simulink model "ALFlight3Wing"  (R2019a)
settings: Solver=VariableStepAuto  StartTime=0.0  StopTime=100  RelTol=1e-3
InitFcn:
  | Ts=.05
  | load('goodMPC.mat')
  | %load('fault2mpc.mat')
  | global counts
  | counts=0
  | 
  | An=[-0.0220400000000000,0.00142200000000000,0,-32.1700000000000,0,0,0,0,0,0;-0.0575900000000000,-0.394300000000000,871,0,0,0,0,0,0,0;-9.50000000000000e-05,-0.00179300000000000,-0.546800000000000,0,0,0,0,0,0,0;0,0,1,0,0,0,0,0,0,0;0,0,0,0,-0.0639900000000000,0,-1,0.0369100000000000,0,0;0,0,0,0,-2.11100000000000,-0.504800000000000,0.193000000000000,0,0,0;0,0,0,0,0.773200000000000,0.0108700000000000,-0.179400000000000,0,0,0;0,0,0,0,0,1,0,0,0,0;0,0,0,0,0,0,1,0,0,0;0,1,0,0,0,0,0,0,0,0]
  | Bn=[0,1.91000000000000e-05,0,0;-18.5800000000000,0,0,0;-1.20000000000000,0,0,0;0,0,0,0;0,0,0,0.00839000000000000;0,0,0.184800000000000,0.105600000000000;0,0,-0.00869900000000000,-0.459100000000000;0,0,0,0;0,0,0,0;0,0,0,0]
  | 
  | 
  |  set_param('ALFlight3Wing/ConstantA','Value','An')
  |  set_param('ALFlight3Wing/ConstantB','Value','Bn')
model workspace (MAT data in the model file):
  MCOS : class17 (value not decoded)
values from neighbouring files (symbols this model uses):
  Af2 = [-0.02204 -0.05759 -9.5e-05 0 0 0 0 0 0 0 0.001422 -0.3943 ... (100 elements, 10x10)]    [UpdatedWorkspace.mat]    (also in current2.mat; finalWorkspace.mat)
  Bf2 = [0 -18.58 -1.2 0 0 0 0 0 0 0 1.91e-05 0 ... (40 elements, 10x4)]    [UpdatedWorkspace.mat]    (also in current2.mat; finalWorkspace.mat)
  Cn = [1 0 0 0 0 0 0 0 0 0 0 0 ... (40 elements, 4x10)]    [UpdatedWorkspace.mat]    (also in current2.mat; finalWorkspace.mat)
  Dn = [0 0 0 0 0 0 0 0 0 0 0 0 ... (16 elements, 4x4)]    [UpdatedWorkspace.mat]    (also in current2.mat; finalWorkspace.mat)
  p = 15    [calcVar.m]    (also in chanceConstraintProgramming4.m = [norminv(.505),norminv(.6),norminv(.7),norminv(.8),norminv(.; dynamicsEst.m)
undefined symbols (not defined in the file or in its folder): Earth, iA, lastPcov, lastu, lastx, MDscale, mmpc_mvseq, mmpc_state, mmpc_ts, mmpc_u0, mmpc_xseq, mmpc_yseq, MVscale, nCC, nu, nud, nv, ny, nym, RMVscale, RYscale, ts, uoff, WGS84, xoff, Yscale
libraries: mpcsigdimcheck_private x44, simulink_extras x3, mpclib x2, commchan3 x1, aerolibtransform2 x1, aerolibfltsims x1, aerolibanimutils x1
(part 2 of 4)

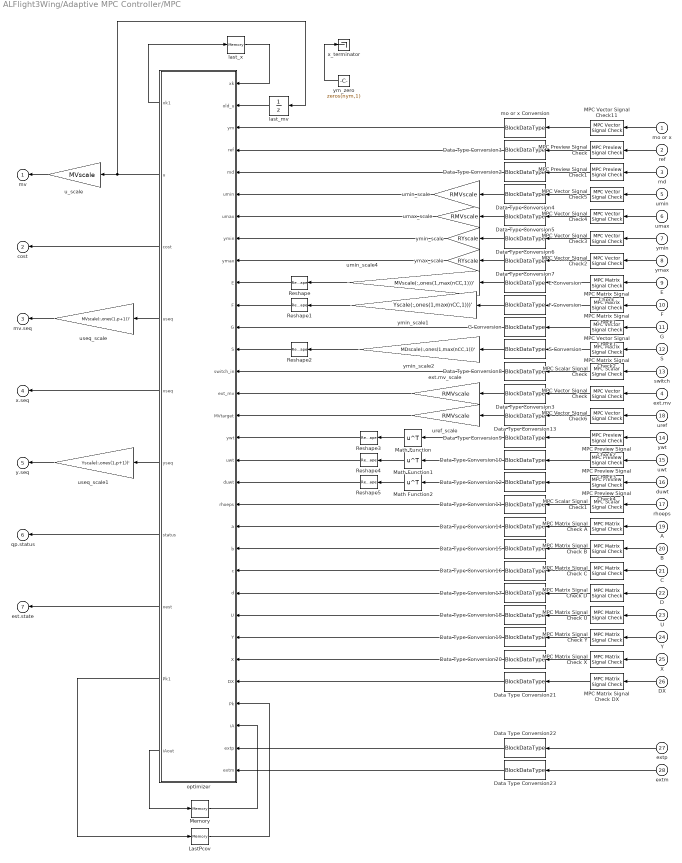
== system ALFlight3Wing/Adaptive MPC Controller/MPC ==
  mo or x : Inport
  ref : Inport  Port=2
  md : Inport  Port=3
  ext.mv : Inport  Port=4
  umin : Inport  Port=5
  umax : Inport  Port=6
  ymin : Inport  Port=7
  ymax : Inport  Port=8
  E : Inport  Port=9
  F : Inport  Port=10
  G : Inport  Port=11
  S : Inport  Port=12
  switch : Inport  Port=13
  ywt : Inport  Port=14
  uwt : Inport  Port=15
  duwt : Inport  Port=16
  rhoeps : Inport  Port=17
  uref : Inport  Port=18
  A : Inport  Port=19
  B : Inport  Port=20
  C : Inport  Port=21
  D : Inport  Port=22
  U : Inport  Port=23
  Y : Inport  Port=24
  X : Inport  Port=25
  DX : Inport  Port=26
  extp : Inport  Port=27
  extm : Inport  Port=28
  Data Type Conversion{1..23} (23 alike) : DataTypeConversion  OutDataTypeStr=BlockDataType
  E Conversion : DataTypeConversion  OutDataTypeStr=BlockDataType
  F Conversion : DataTypeConversion  OutDataTypeStr=BlockDataType
  G Conversion : DataTypeConversion  OutDataTypeStr=BlockDataType
  LastPcov : Memory  InitialCondition=lastPcov  InheritSampleTime=on  LinearizeAsDelay=on
  MPC Matrix Signal Check : mpcsigdimcheck_private/MPC Matrix Signal Check  blockname=blk  signalname='CustomConstraint.E'  numrow=max(nCC,1)  numcol=nu  steps=0  isLTV=0
      settings: SourceProductName=MATLAB Runtime - Model Predictive Control Toolbox Addin  SourceProductBaseCode=Missing
  MPC Matrix Signal Check A : mpcsigdimcheck_private/MPC Matrix Signal Check  blockname=blk  signalname='Model.A'  numrow=nxp  numcol=nxp  steps=p  isLTV=isLTV
      settings: SourceProductName=MATLAB Runtime - Model Predictive Control Toolbox Addin  SourceProductBaseCode=Missing
  MPC Matrix Signal Check B : mpcsigdimcheck_private/MPC Matrix Signal Check  blockname=blk  signalname='Model.B'  numrow=nxp  numcol=nu+nv-1+nud  steps=p  isLTV=isLTV
      settings: SourceProductName=MATLAB Runtime - Model Predictive Control Toolbox Addin  SourceProductBaseCode=Missing
  MPC Matrix Signal Check C : mpcsigdimcheck_private/MPC Matrix Signal Check  blockname=blk  signalname='Model.C'  numrow=ny  numcol=nxp  steps=p  isLTV=isLTV
      settings: SourceProductName=MATLAB Runtime - Model Predictive Control Toolbox Addin  SourceProductBaseCode=Missing
  MPC Matrix Signal Check D : mpcsigdimcheck_private/MPC Matrix Signal Check  blockname=blk  signalname='Model.D'  numrow=ny  numcol=nu+nv-1+nud  steps=p  isLTV=isLTV
      settings: SourceProductName=MATLAB Runtime - Model Predictive Control Toolbox Addin  SourceProductBaseCode=Missing
  MPC Matrix Signal Check DX : mpcsigdimcheck_private/MPC Matrix Signal Check  blockname=blk  signalname='Model.DX'  numrow=nxp  numcol=1  steps=p  isLTV=isLTV
      settings: SourceProductName=MATLAB Runtime - Model Predictive Control Toolbox Addin  SourceProductBaseCode=Missing
  MPC Matrix Signal Check U : mpcsigdimcheck_private/MPC Matrix Signal Check  blockname=blk  signalname='Model.U'  numrow=nu+nv-1+nud  numcol=1  steps=p  isLTV=isLTV
      settings: SourceProductName=MATLAB Runtime - Model Predictive Control Toolbox Addin  SourceProductBaseCode=Missing
  MPC Matrix Signal Check X : mpcsigdimcheck_private/MPC Matrix Signal Check  blockname=blk  signalname='Model.X'  numrow=nxp  numcol=1  steps=p  isLTV=isLTV
      settings: SourceProductName=MATLAB Runtime - Model Predictive Control Toolbox Addin  SourceProductBaseCode=Missing
  MPC Matrix Signal Check Y : mpcsigdimcheck_private/MPC Matrix Signal Check  blockname=blk  signalname='Model.Y'  numrow=ny  numcol=1  steps=p  isLTV=isLTV
      settings: SourceProductName=MATLAB Runtime - Model Predictive Control Toolbox Addin  SourceProductBaseCode=Missing
  MPC Matrix Signal Check1 : mpcsigdimcheck_private/MPC Matrix Signal Check  blockname=blk  signalname='CustomConstraint.F'  numrow=max(nCC,1)  numcol=ny  steps=0  isLTV=0
      settings: SourceProductName=MATLAB Runtime - Model Predictive Control Toolbox Addin  SourceProductBaseCode=Missing
  MPC Matrix Signal Check2 : mpcsigdimcheck_private/MPC Matrix Signal Check  blockname=blk  signalname='CustomConstraint.S'  numrow=max(nCC,1)  numcol=max(nv-1,1)  steps=0  isLTV=0
      settings: SourceProductName=MATLAB Runtime - Model Predictive Control Toolbox Addin  SourceProductBaseCode=Missing
  MPC Preview Signal Check : mpcsigdimcheck_private/MPC Preview Signal Check  blockname=blk  signalname='ref'  numrow=p  numcol=ny
      settings: SourceProductName=MATLAB Runtime - Model Predictive Control Toolbox Addin  SourceProductBaseCode=Missing
  MPC Preview Signal Check1 : mpcsigdimcheck_private/MPC Preview Signal Check  blockname=blk  signalname='md'  numrow=p+1  numcol=max(nv-1,1)
      settings: SourceProductName=MATLAB Runtime - Model Predictive Control Toolbox Addin  SourceProductBaseCode=Missing
  MPC Preview Signal Check2 : mpcsigdimcheck_private/MPC Preview Signal Check  blockname=blk  signalname='y.wt'  numrow=p  numcol=ny
      settings: SourceProductName=MATLAB Runtime - Model Predictive Control Toolbox Addin  SourceProductBaseCode=Missing
  MPC Preview Signal Check3 : mpcsigdimcheck_private/MPC Preview Signal Check  blockname=blk  signalname='u.wt'  numrow=p  numcol=nu
      settings: SourceProductName=MATLAB Runtime - Model Predictive Control Toolbox Addin  SourceProductBaseCode=Missing
  MPC Preview Signal Check4 : mpcsigdimcheck_private/MPC Preview Signal Check  blockname=blk  signalname='du.wt'  numrow=p  numcol=nu
      settings: SourceProductName=MATLAB Runtime - Model Predictive Control Toolbox Addin  SourceProductBaseCode=Missing
  MPC Scalar Signal Check : mpcsigdimcheck_private/MPC Scalar Signal Check  blockname=blk  signalname='switch'
      settings: SourceProductName=MATLAB Runtime - Model Predictive Control Toolbox Addin  SourceProductBaseCode=Missing
  MPC Scalar Signal Check1 : mpcsigdimcheck_private/MPC Scalar Signal Check  blockname=blk  signalname='ecr.wt'
      settings: SourceProductName=MATLAB Runtime - Model Predictive Control Toolbox Addin  SourceProductBaseCode=Missing
  MPC Vector Signal Check : mpcsigdimcheck_private/MPC Vector Signal Check  blockname=blk  signalname='ext.mv'  num=nu  vectortype=Any
      settings: SourceProductName=MATLAB Runtime - Model Predictive Control Toolbox Addin  SourceProductBaseCode=Missing
  MPC Vector Signal Check1 : mpcsigdimcheck_private/MPC Vector Signal Check  blockname=blk  signalname='CustomConstraint.G'  num=max(nCC,1)  vectortype=Column
      settings: SourceProductName=MATLAB Runtime - Model Predictive Control Toolbox Addin  SourceProductBaseCode=Missing
  MPC Vector Signal Check11 : mpcsigdimcheck_private/MPC Vector Signal Check  blockname=blk  signalname=strmoorx  num=nmoorx  vectortype=Any
      settings: SourceProductName=MATLAB Runtime - Model Predictive Control Toolbox Addin  SourceProductBaseCode=Missing
  MPC Vector Signal Check2 : mpcsigdimcheck_private/MPC Vector Signal Check  blockname=blk  signalname='ymax'  num=ny  vectortype=Any
      settings: SourceProductName=MATLAB Runtime - Model Predictive Control Toolbox Addin  SourceProductBaseCode=Missing
  MPC Vector Signal Check3 : mpcsigdimcheck_private/MPC Vector Signal Check  blockname=blk  signalname='ymin'  num=ny  vectortype=Any
      settings: SourceProductName=MATLAB Runtime - Model Predictive Control Toolbox Addin  SourceProductBaseCode=Missing
  MPC Vector Signal Check4 : mpcsigdimcheck_private/MPC Vector Signal Check  blockname=blk  signalname='umax'  num=nu  vectortype=Any
      settings: SourceProductName=MATLAB Runtime - Model Predictive Control Toolbox Addin  SourceProductBaseCode=Missing
  MPC Vector Signal Check5 : mpcsigdimcheck_private/MPC Vector Signal Check  blockname=blk  signalname='umin'  num=nu  vectortype=Any
      settings: SourceProductName=MATLAB Runtime - Model Predictive Control Toolbox Addin  SourceProductBaseCode=Missing
  MPC Vector Signal Check6 : mpcsigdimcheck_private/MPC Vector Signal Check  blockname=blk  signalname='mv.target'  num=nu  vectortype=Any
      settings: SourceProductName=MATLAB Runtime - Model Predictive Control Toolbox Addin  SourceProductBaseCode=Missing
  Math Function : Math  Operator=transpose  SaturateOnIntegerOverflow=on
  Math Function1 : Math  Operator=transpose  SaturateOnIntegerOverflow=on
  Math Function2 : Math  Operator=transpose  SaturateOnIntegerOverflow=on
  Memory : Memory  InitialCondition=iA  InheritSampleTime=on  LinearizeAsDelay=on
  Reshape : Reshape  OutputDimensionality=Customize  OutputDimensions=double([max(nCC,1),nu])
  Reshape1 : Reshape  OutputDimensionality=Customize  OutputDimensions=double([max(nCC,1),ny])
  Reshape2 : Reshape  OutputDimensionality=Customize  OutputDimensions=double([max(nCC,1),max(nv-1,1)])
  Reshape3 : Reshape  OutputDimensionality=Column vector (2-D)
  Reshape4 : Reshape  OutputDimensionality=Column vector (2-D)
  Reshape5 : Reshape  OutputDimensionality=Column vector (2-D)
  S Conversion : DataTypeConversion  OutDataTypeStr=BlockDataType
  ext.mv_scale : Gain  Gain=RMVscale  SampleTime=ts
  last_mv : UnitDelay  InitialCondition=lastu+uoff  SampleTime=ts  HasFrameUpgradeWarning=on
  last_x : Memory  InitialCondition=lastx+xoff  InheritSampleTime=on  LinearizeAsDelay=on
  mo or x Conversion : DataTypeConversion  OutDataTypeStr=BlockDataType
  optimizer : Subsystem  VariantControlMode=Label  Variant=on  VariantControl=Variant1  LabelModeActiveChoice=FixedHorizon
  u_scale : Gain  Gain=MVscale  SampleTime=ts
  umax_scale : Gain  Gain=RMVscale  SampleTime=ts
  umin_scale : Gain  Gain=RMVscale  SampleTime=ts
  umin_scale4 : Gain  Gain=MVscale(:,ones(1,max(nCC,1)))'  SampleTime=ts
  uref_scale : Gain  Gain=RMVscale  SampleTime=ts
  useq_scale : Gain  Gain=MVscale(:,ones(1,p+1))'  SampleTime=ts
  useq_scale1 : Gain  Gain=Yscale(:,ones(1,p+1))'  SampleTime=ts
  x_terminator : Terminator
  ym_zero : Constant  Value=zeros(nym,1)  OutDataTypeStr=BlockDataType
  ymax_scale : Gain  Gain=RYscale  SampleTime=ts
  ymin_scale : Gain  Gain=RYscale  SampleTime=ts
  ymin_scale1 : Gain  Gain=Yscale(:,ones(1,max(nCC,1)))'  SampleTime=ts
  ymin_scale2 : Gain  Gain=MDscale(:,ones(1,max(nCC,1)))'  SampleTime=ts
  mv : Outport  OutDataTypeStr=BlockDataType
  cost : Outport  Port=2  OutDataTypeStr=BlockDataType
  mv.seq : Outport  Port=3  OutDataTypeStr=BlockDataType
  x.seq : Outport  Port=4  OutDataTypeStr=BlockDataType
  y.seq : Outport  Port=5  OutDataTypeStr=BlockDataType
  qp.status : Outport  Port=6  OutDataTypeStr=BlockDataType
  est.state : Outport  Port=7  OutDataTypeStr=BlockDataType
  wires:
  extm/1 -> Data Type Conversion23/1
  extp/1 -> Data Type Conversion22/1
  Data Type Conversion23/1 -> optimizer/32(extm)
  Data Type Conversion22/1 -> optimizer/31(extp)
  optimizer/10(" iAout") -> Memory/1
  optimizer/9(" Pk1") -> LastPcov/1
  optimizer/8(" xest") -> est.state/1
  optimizer/7(" status") -> qp.status/1
  optimizer/6(" yseq") -> useq_scale1/1
  optimizer/5(" xseq") -> x.seq/1
  optimizer/4(" useq") -> useq_scale/1
  optimizer/3(" cost") -> cost/1
  optimizer/2(" u") -> last_mv/1, u_scale/1
  optimizer/1(" xk1") -> last_x/1
  Memory/1 -> optimizer/30("iA ")
  LastPcov/1 -> optimizer/29("Pk ")
  Data Type Conversion21/1 -> optimizer/28("DX ")
  Data Type Conversion20/1 -> optimizer/27("X ")
  Data Type Conversion19/1 -> optimizer/26("Y ")
  Data Type Conversion18/1 -> optimizer/25("U ")
  Data Type Conversion17/1 -> optimizer/24("d ")
  Data Type Conversion16/1 -> optimizer/23("c ")
  Data Type Conversion15/1 -> optimizer/22("b ")
  Data Type Conversion14/1 -> optimizer/21("a ")
  Data Type Conversion11/1 -> optimizer/20("rhoeps ")
  Reshape5/1 -> optimizer/19("duwt ")
  Reshape4/1 -> optimizer/18("uwt ")
  Reshape3/1 -> optimizer/17("ywt ")
  uref_scale/1 -> optimizer/16("MVtarget ")
  ext.mv_scale/1 -> optimizer/15("ext_mv ")
  Data Type Conversion8/1 -> optimizer/14("switch_in ")
  Reshape2/1 -> optimizer/13("S ")
  G Conversion/1 -> optimizer/12("G ")
  Reshape1/1 -> optimizer/11("F ")
  Reshape/1 -> optimizer/10("E ")
  ymax_scale/1 -> optimizer/9("ymax ")
  ymin_scale/1 -> optimizer/8("ymin ")
  umax_scale/1 -> optimizer/7("umax ")
  umin_scale/1 -> optimizer/6("umin ")
  Data Type Conversion2/1 -> optimizer/5("md ")
  Data Type Conversion1/1 -> optimizer/4("ref ")
  mo or x Conversion/1 -> optimizer/3("ym ")
  last_mv/1 -> optimizer/2("old_u ")
  last_x/1 -> optimizer/1("xk ")
  useq_scale1/1 -> y.seq/1
  Math Function2/1 -> Reshape5/1
  Math Function1/1 -> Reshape4/1
  Math Function/1 -> Reshape3/1
  MPC Matrix Signal Check1/1 -> F Conversion/1
  umin_scale4/1 -> Reshape/1
  ymin_scale1/1 -> Reshape1/1
  G/1 -> MPC Vector Signal Check1/1
  F/1 -> MPC Matrix Signal Check1/1
  E Conversion/1 -> umin_scale4/1
  ymin_scale2/1 -> Reshape2/1
  MPC Matrix Signal Check/1 -> E Conversion/1
  S/1 -> MPC Matrix Signal Check2/1
  E/1 -> MPC Matrix Signal Check/1
  MPC Matrix Signal Check2/1 -> S Conversion/1
  MPC Vector Signal Check1/1 -> G Conversion/1
  S Conversion/1 -> ymin_scale2/1
  F Conversion/1 -> ymin_scale1/1
  MPC Matrix Signal Check DX/1 -> Data Type Conversion21/1
  MPC Matrix Signal Check X/1 -> Data Type Conversion20/1
  MPC Matrix Signal Check Y/1 -> Data Type Conversion19/1
  MPC Matrix Signal Check U/1 -> Data Type Conversion18/1
  MPC Matrix Signal Check D/1 -> Data Type Conversion17/1
  MPC Matrix Signal Check C/1 -> Data Type Conversion16/1
  MPC Matrix Signal Check B/1 -> Data Type Conversion15/1
  MPC Matrix Signal Check A/1 -> Data Type Conversion14/1
  MPC Scalar Signal Check1/1 -> Data Type Conversion11/1
  MPC Preview Signal Check4/1 -> Data Type Conversion12/1
  MPC Preview Signal Check3/1 -> Data Type Conversion10/1
  MPC Preview Signal Check2/1 -> Data Type Conversion9/1
  MPC Vector Signal Check6/1 -> Data Type Conversion13/1
  MPC Vector Signal Check/1 -> Data Type Conversion3/1
  MPC Scalar Signal Check/1 -> Data Type Conversion8/1
  MPC Vector Signal Check2/1 -> Data Type Conversion7/1
  MPC Vector Signal Check3/1 -> Data Type Conversion6/1
  MPC Vector Signal Check4/1 -> Data Type Conversion5/1
  MPC Vector Signal Check5/1 -> Data Type Conversion4/1
  MPC Preview Signal Check1/1 -> Data Type Conversion2/1
  MPC Preview Signal Check/1 -> Data Type Conversion1/1
  MPC Vector Signal Check11/1 -> mo or x Conversion/1
  useq_scale/1 -> mv.seq/1
  u_scale/1 -> mv/1
  DX/1 -> MPC Matrix Signal Check DX/1
  X/1 -> MPC Matrix Signal Check X/1
  Y/1 -> MPC Matrix Signal Check Y/1
  U/1 -> MPC Matrix Signal Check U/1
  D/1 -> MPC Matrix Signal Check D/1
  C/1 -> MPC Matrix Signal Check C/1
  B/1 -> MPC Matrix Signal Check B/1
  A/1 -> MPC Matrix Signal Check A/1
  md/1 -> MPC Preview Signal Check1/1
  umin/1 -> MPC Vector Signal Check5/1
  umax/1 -> MPC Vector Signal Check4/1
  ymin/1 -> MPC Vector Signal Check3/1
  ymax/1 -> MPC Vector Signal Check2/1
  switch/1 -> MPC Scalar Signal Check/1
  ext.mv/1 -> MPC Vector Signal Check/1
  Data Type Conversion3/1 -> ext.mv_scale/1
  ref/1 -> MPC Preview Signal Check/1
  mo or x/1 -> MPC Vector Signal Check11/1
  ywt/1 -> MPC Preview Signal Check2/1
  uwt/1 -> MPC Preview Signal Check3/1
  Data Type Conversion4/1 -> umin_scale/1
  Data Type Conversion5/1 -> umax_scale/1
  Data Type Conversion7/1 -> ymax_scale/1
  Data Type Conversion9/1 -> Math Function/1
  Data Type Conversion12/1 -> Math Function2/1
  Data Type Conversion6/1 -> ymin_scale/1
  rhoeps/1 -> MPC Scalar Signal Check1/1
  duwt/1 -> MPC Preview Signal Check4/1
  Data Type Conversion10/1 -> Math Function1/1
  uref/1 -> MPC Vector Signal Check6/1
  Data Type Conversion13/1 -> uref_scale/1
  ym_zero/1 -> x_terminator/1

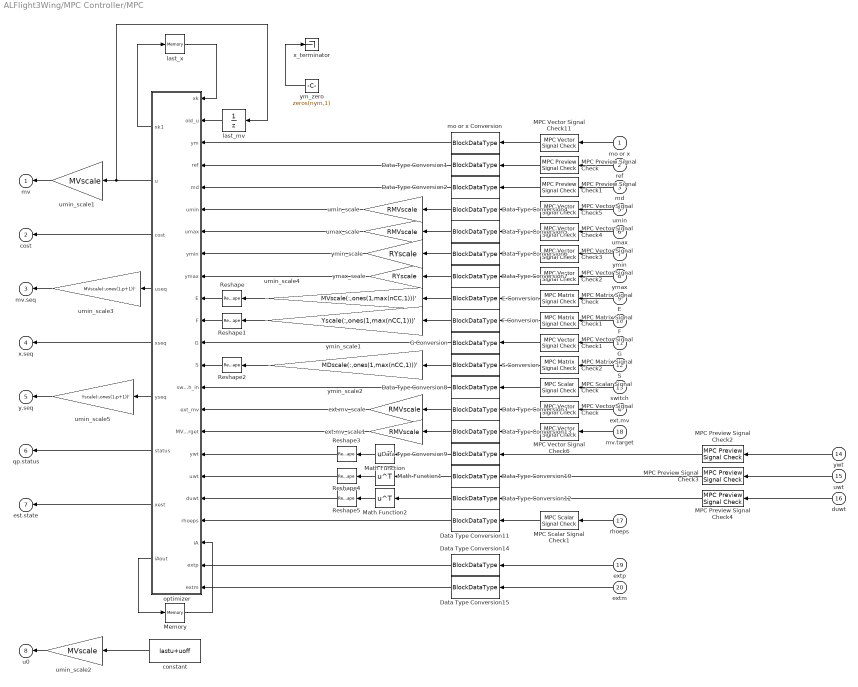
== system ALFlight3Wing/MPC Controller/MPC ==
  mo or x : Inport
  ref : Inport  Port=2
  md : Inport  Port=3
  ext.mv : Inport  Port=4
  umin : Inport  Port=5
  umax : Inport  Port=6
  ymin : Inport  Port=7
  ymax : Inport  Port=8
  E : Inport  Port=9
  F : Inport  Port=10
  G : Inport  Port=11
  S : Inport  Port=12
  switch : Inport  Port=13
  ywt : Inport  Port=14
  uwt : Inport  Port=15
  duwt : Inport  Port=16
  rhoeps : Inport  Port=17
  mv.target : Inport  Port=18
  extp : Inport  Port=19
  extm : Inport  Port=20
  Data Type Conversion{1..15} (15 alike) : DataTypeConversion  OutDataTypeStr=BlockDataType
  E Conversion : DataTypeConversion  OutDataTypeStr=BlockDataType
  F Conversion : DataTypeConversion  OutDataTypeStr=BlockDataType
  G Conversion : DataTypeConversion  OutDataTypeStr=BlockDataType
  MPC Matrix Signal Check : mpcsigdimcheck_private/MPC Matrix Signal Check  blockname=blk  signalname='CustomConstraint.E'  numrow=max(nCC,1)  numcol=nu  steps=0  isLTV=0
      settings: SourceProductName=MATLAB Runtime - Model Predictive Control Toolbox Addin  SourceProductBaseCode=Missing
  MPC Matrix Signal Check1 : mpcsigdimcheck_private/MPC Matrix Signal Check  blockname=blk  signalname='CustomConstraint.F'  numrow=max(nCC,1)  numcol=ny  steps=0  isLTV=0
      settings: SourceProductName=MATLAB Runtime - Model Predictive Control Toolbox Addin  SourceProductBaseCode=Missing
  MPC Matrix Signal Check2 : mpcsigdimcheck_private/MPC Matrix Signal Check  blockname=blk  signalname='CustomConstraint.S'  numrow=max(nCC,1)  numcol=max(nv-1,1)  steps=0  isLTV=0
      settings: SourceProductName=MATLAB Runtime - Model Predictive Control Toolbox Addin  SourceProductBaseCode=Missing
  MPC Preview Signal Check : mpcsigdimcheck_private/MPC Preview Signal Check  blockname=blk  signalname='ref'  numrow=p  numcol=ny
      settings: SourceProductName=MATLAB Runtime - Model Predictive Control Toolbox Addin  SourceProductBaseCode=Missing
  MPC Preview Signal Check1 : mpcsigdimcheck_private/MPC Preview Signal Check  blockname=blk  signalname='md'  numrow=p+1  numcol=max(nv-1,1)
      settings: SourceProductName=MATLAB Runtime - Model Predictive Control Toolbox Addin  SourceProductBaseCode=Missing
  MPC Preview Signal Check2 : mpcsigdimcheck_private/MPC Preview Signal Check  blockname=blk  signalname='y.wt'  numrow=p  numcol=ny
      settings: SourceProductName=MATLAB Runtime - Model Predictive Control Toolbox Addin  SourceProductBaseCode=Missing
  MPC Preview Signal Check3 : mpcsigdimcheck_private/MPC Preview Signal Check  blockname=blk  signalname='u.wt'  numrow=p  numcol=nu
      settings: SourceProductName=MATLAB Runtime - Model Predictive Control Toolbox Addin  SourceProductBaseCode=Missing
  MPC Preview Signal Check4 : mpcsigdimcheck_private/MPC Preview Signal Check  blockname=blk  signalname='du.wt'  numrow=p  numcol=nu
      settings: SourceProductName=MATLAB Runtime - Model Predictive Control Toolbox Addin  SourceProductBaseCode=Missing
  MPC Scalar Signal Check : mpcsigdimcheck_private/MPC Scalar Signal Check  blockname=blk  signalname='switch'
      settings: SourceProductName=MATLAB Runtime - Model Predictive Control Toolbox Addin  SourceProductBaseCode=Missing
  MPC Scalar Signal Check1 : mpcsigdimcheck_private/MPC Scalar Signal Check  blockname=blk  signalname='ecr.wt'
      settings: SourceProductName=MATLAB Runtime - Model Predictive Control Toolbox Addin  SourceProductBaseCode=Missing
  MPC Vector Signal Check : mpcsigdimcheck_private/MPC Vector Signal Check  blockname=blk  signalname='ext.mv'  num=nu  vectortype=Any
      settings: SourceProductName=MATLAB Runtime - Model Predictive Control Toolbox Addin  SourceProductBaseCode=Missing
  MPC Vector Signal Check1 : mpcsigdimcheck_private/MPC Vector Signal Check  blockname=blk  signalname='CustomConstraint.G'  num=max(nCC,1)  vectortype=Column
      settings: SourceProductName=MATLAB Runtime - Model Predictive Control Toolbox Addin  SourceProductBaseCode=Missing
  MPC Vector Signal Check11 : mpcsigdimcheck_private/MPC Vector Signal Check  blockname=blk  signalname=strmoorx  num=nmoorx  vectortype=Any
      settings: SourceProductName=MATLAB Runtime - Model Predictive Control Toolbox Addin  SourceProductBaseCode=Missing
  MPC Vector Signal Check2 : mpcsigdimcheck_private/MPC Vector Signal Check  blockname=blk  signalname='ymax'  num=ny  vectortype=Any
      settings: SourceProductName=MATLAB Runtime - Model Predictive Control Toolbox Addin  SourceProductBaseCode=Missing
  MPC Vector Signal Check3 : mpcsigdimcheck_private/MPC Vector Signal Check  blockname=blk  signalname='ymin'  num=ny  vectortype=Any
      settings: SourceProductName=MATLAB Runtime - Model Predictive Control Toolbox Addin  SourceProductBaseCode=Missing
  MPC Vector Signal Check4 : mpcsigdimcheck_private/MPC Vector Signal Check  blockname=blk  signalname='umax'  num=nu  vectortype=Any
      settings: SourceProductName=MATLAB Runtime - Model Predictive Control Toolbox Addin  SourceProductBaseCode=Missing
  MPC Vector Signal Check5 : mpcsigdimcheck_private/MPC Vector Signal Check  blockname=blk  signalname='umin'  num=nu  vectortype=Any
      settings: SourceProductName=MATLAB Runtime - Model Predictive Control Toolbox Addin  SourceProductBaseCode=Missing
  MPC Vector Signal Check6 : mpcsigdimcheck_private/MPC Vector Signal Check  blockname=blk  signalname='mv.target'  num=nu  vectortype=Any
      settings: SourceProductName=MATLAB Runtime - Model Predictive Control Toolbox Addin  SourceProductBaseCode=Missing
  Math Function : Math  Operator=transpose  SaturateOnIntegerOverflow=on
  Math Function1 : Math  Operator=transpose  SaturateOnIntegerOverflow=on
  Math Function2 : Math  Operator=transpose  SaturateOnIntegerOverflow=on
  Memory : Memory  InitialCondition=iA  InheritSampleTime=on  LinearizeAsDelay=on
  Reshape : Reshape  OutputDimensionality=Customize  OutputDimensions=double([max(nCC,1),nu])
  Reshape1 : Reshape  OutputDimensionality=Customize  OutputDimensions=double([max(nCC,1),ny])
  Reshape2 : Reshape  OutputDimensionality=Customize  OutputDimensions=double([max(nCC,1),max(nv-1,1)])
  Reshape3 : Reshape  OutputDimensionality=Column vector (2-D)
  Reshape4 : Reshape  OutputDimensionality=Column vector (2-D)
  Reshape5 : Reshape  OutputDimensionality=Column vector (2-D)
  S Conversion : DataTypeConversion  OutDataTypeStr=BlockDataType
  constant : Constant  Value=lastu+uoff
  ext.mv_scale : Gain  Gain=RMVscale  SampleTime=ts
  ext.mv_scale1 : Gain  Gain=RMVscale  SampleTime=ts
  last_mv : UnitDelay  InitialCondition=lastu+uoff  SampleTime=ts  HasFrameUpgradeWarning=on
  last_x : Memory  InitialCondition=lastx+xoff  InheritSampleTime=on  LinearizeAsDelay=on
  mo or x Conversion : DataTypeConversion  OutDataTypeStr=BlockDataType
  optimizer : Subsystem  VariantControlMode=Label  Variant=on  VariantControl=Variant1  LabelModeActiveChoice=FixedHorizon
  umax_scale : Gain  Gain=RMVscale  SampleTime=ts
  umin_scale : Gain  Gain=RMVscale  SampleTime=ts
  umin_scale1 : Gain  Gain=MVscale  SampleTime=ts
  umin_scale2 : Gain  Gain=MVscale  SampleTime=ts
  umin_scale3 : Gain  Gain=MVscale(:,ones(1,p+1))'  SampleTime=ts
  umin_scale4 : Gain  Gain=MVscale(:,ones(1,max(nCC,1)))'  SampleTime=ts
  umin_scale5 : Gain  Gain=Yscale(:,ones(1,p+1))'  SampleTime=ts
  x_terminator : Terminator
  ym_zero : Constant  Value=zeros(nym,1)  OutDataTypeStr=BlockDataType
  ymax_scale : Gain  Gain=RYscale  SampleTime=ts
  ymin_scale : Gain  Gain=RYscale  SampleTime=ts
  ymin_scale1 : Gain  Gain=Yscale(:,ones(1,max(nCC,1)))'  SampleTime=ts
  ymin_scale2 : Gain  Gain=MDscale(:,ones(1,max(nCC,1)))'  SampleTime=ts
  mv : Outport  OutDataTypeStr=BlockDataType
  cost : Outport  Port=2  OutDataTypeStr=BlockDataType
  mv.seq : Outport  Port=3  OutDataTypeStr=BlockDataType
  x.seq : Outport  Port=4  OutDataTypeStr=BlockDataType
  y.seq : Outport  Port=5  OutDataTypeStr=BlockDataType
  qp.status : Outport  Port=6  OutDataTypeStr=BlockDataType
  est.state : Outport  Port=7  OutDataTypeStr=BlockDataType
  u0 : Outport  Port=8  OutDataTypeStr=BlockDataType
  wires:
  extm/1 -> Data Type Conversion15/1
  extp/1 -> Data Type Conversion14/1
  Data Type Conversion14/1 -> optimizer/22(extp)
  Data Type Conversion15/1 -> optimizer/23(extm)
  optimizer/9(" iAout") -> Memory/1
  optimizer/8(" xest") -> est.state/1
  optimizer/7(" status") -> qp.status/1
  optimizer/6(" yseq") -> umin_scale5/1
  optimizer/5(" xseq") -> x.seq/1
  optimizer/4(" useq") -> umin_scale3/1
  optimizer/3(" cost") -> cost/1
  optimizer/2(" u") -> umin_scale1/1, last_mv/1
  optimizer/1(" xk1") -> last_x/1
  Memory/1 -> optimizer/21("iA ")
  Data Type Conversion11/1 -> optimizer/20("rhoeps ")
  Reshape5/1 -> optimizer/19("duwt ")
  Reshape4/1 -> optimizer/18("uwt ")
  Reshape3/1 -> optimizer/17("ywt ")
  ext.mv_scale1/1 -> optimizer/16("MVtarget ")
  ext.mv_scale/1 -> optimizer/15("ext_mv ")
  Data Type Conversion8/1 -> optimizer/14("switch_in ")
  Reshape2/1 -> optimizer/13("S ")
  G Conversion/1 -> optimizer/12("G ")
  Reshape1/1 -> optimizer/11("F ")
  Reshape/1 -> optimizer/10("E ")
  ymax_scale/1 -> optimizer/9("ymax ")
  ymin_scale/1 -> optimizer/8("ymin ")
  umax_scale/1 -> optimizer/7("umax ")
  umin_scale/1 -> optimizer/6("umin ")
  Data Type Conversion2/1 -> optimizer/5("md ")
  Data Type Conversion1/1 -> optimizer/4("ref ")
  mo or x Conversion/1 -> optimizer/3("ym ")
  last_mv/1 -> optimizer/2("old_u ")
  last_x/1 -> optimizer/1("xk ")
  umin_scale5/1 -> y.seq/1
  Math Function2/1 -> Reshape5/1
  Math Function1/1 -> Reshape4/1
  Math Function/1 -> Reshape3/1
  ymin_scale2/1 -> Reshape2/1
  ymin_scale1/1 -> Reshape1/1
  umin_scale4/1 -> Reshape/1
  S Conversion/1 -> ymin_scale2/1
  F Conversion/1 -> ymin_scale1/1
  E Conversion/1 -> umin_scale4/1
  MPC Matrix Signal Check/1 -> E Conversion/1
  MPC Matrix Signal Check1/1 -> F Conversion/1
  MPC Vector Signal Check1/1 -> G Conversion/1
  MPC Matrix Signal Check2/1 -> S Conversion/1
  S/1 -> MPC Matrix Signal Check2/1
  G/1 -> MPC Vector Signal Check1/1
  F/1 -> MPC Matrix Signal Check1/1
  E/1 -> MPC Matrix Signal Check/1
  MPC Preview Signal Check1/1 -> Data Type Conversion2/1
  MPC Preview Signal Check/1 -> Data Type Conversion1/1
  MPC Vector Signal Check11/1 -> mo or x Conversion/1
  MPC Scalar Signal Check1/1 -> Data Type Conversion11/1
  MPC Preview Signal Check4/1 -> Data Type Conversion12/1
  MPC Preview Signal Check3/1 -> Data Type Conversion10/1
  MPC Preview Signal Check2/1 -> Data Type Conversion9/1
  MPC Vector Signal Check6/1 -> Data Type Conversion13/1
  MPC Vector Signal Check5/1 -> Data Type Conversion4/1
  MPC Vector Signal Check4/1 -> Data Type Conversion5/1
  MPC Vector Signal Check3/1 -> Data Type Conversion6/1
  MPC Vector Signal Check2/1 -> Data Type Conversion7/1
  MPC Scalar Signal Check/1 -> Data Type Conversion8/1
  MPC Vector Signal Check/1 -> Data Type Conversion3/1
  ym_zero/1 -> x_terminator/1
  umin_scale3/1 -> mv.seq/1
  umin_scale1/1 -> mv/1
  umin_scale2/1 -> u0/1
  constant/1 -> umin_scale2/1
  Data Type Conversion13/1 -> ext.mv_scale1/1
  mv.target/1 -> MPC Vector Signal Check6/1
  Data Type Conversion10/1 -> Math Function1/1
  duwt/1 -> MPC Preview Signal Check4/1
  rhoeps/1 -> MPC Scalar Signal Check1/1
  Data Type Conversion6/1 -> ymin_scale/1
  Data Type Conversion12/1 -> Math Function2/1
  Data Type Conversion9/1 -> Math Function/1
  Data Type Conversion7/1 -> ymax_scale/1
  Data Type Conversion5/1 -> umax_scale/1
  Data Type Conversion4/1 -> umin_scale/1
  uwt/1 -> MPC Preview Signal Check3/1
  ywt/1 -> MPC Preview Signal Check2/1
  mo or x/1 -> MPC Vector Signal Check11/1
  ref/1 -> MPC Preview Signal Check/1
  Data Type Conversion3/1 -> ext.mv_scale/1
  ext.mv/1 -> MPC Vector Signal Check/1
  switch/1 -> MPC Scalar Signal Check/1
  ymax/1 -> MPC Vector Signal Check2/1
  ymin/1 -> MPC Vector Signal Check3/1
  umax/1 -> MPC Vector Signal Check4/1
  umin/1 -> MPC Vector Signal Check5/1
  md/1 -> MPC Preview Signal Check1/1

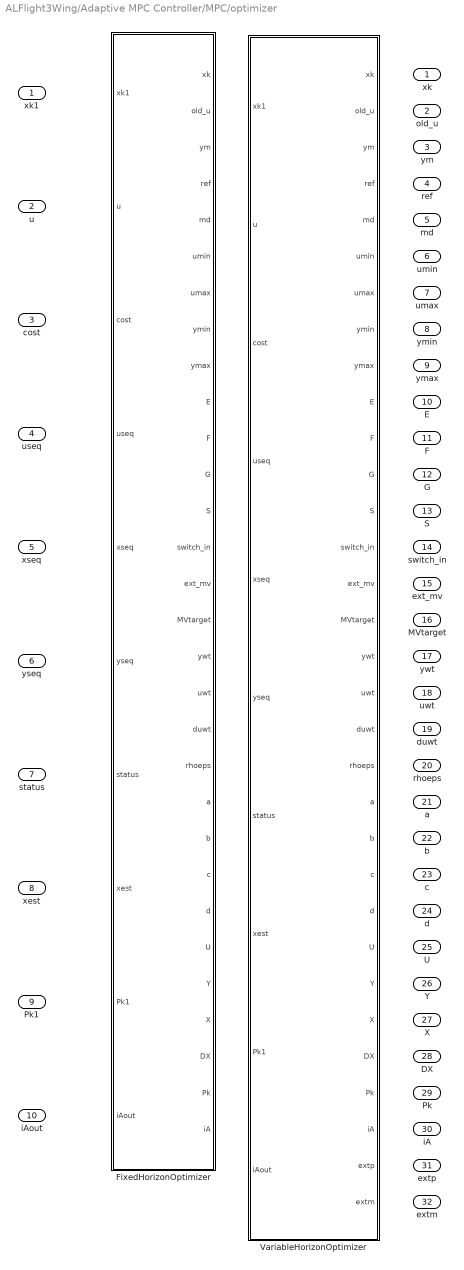
== system ALFlight3Wing/Adaptive MPC Controller/MPC/optimizer ==
  "xk " : Inport
  "old_u " : Inport  Port=2
  "ym " : Inport  Port=3
  "ref " : Inport  Port=4
  "md " : Inport  Port=5
  "umin " : Inport  Port=6
  "umax " : Inport  Port=7
  "ymin " : Inport  Port=8
  "ymax " : Inport  Port=9
  "E " : Inport  Port=10
  "F " : Inport  Port=11
  "G " : Inport  Port=12
  "S " : Inport  Port=13
  "switch_in " : Inport  Port=14
  "ext_mv " : Inport  Port=15
  "MVtarget " : Inport  Port=16
  "ywt " : Inport  Port=17
  "uwt " : Inport  Port=18
  "duwt " : Inport  Port=19
  "rhoeps " : Inport  Port=20
  "a " : Inport  Port=21
  "b " : Inport  Port=22
  "c " : Inport  Port=23
  "d " : Inport  Port=24
  "U " : Inport  Port=25
  "Y " : Inport  Port=26
  "X " : Inport  Port=27
  "DX " : Inport  Port=28
  "Pk " : Inport  Port=29
  "iA " : Inport  Port=30
  extp : Inport  Port=31
  extm : Inport  Port=32
  FixedHorizonOptimizer : MATLAB Function  VariantControl=FixedHorizon
  VariableHorizonOptimizer : MATLAB Function  VariantControl=VariableHorizon
  " xk1" : Outport
  " u" : Outport  Port=2
  " cost" : Outport  Port=3
  " useq" : Outport  Port=4
  " xseq" : Outport  Port=5
  " yseq" : Outport  Port=6
  " status" : Outport  Port=7
  " xest" : Outport  Port=8
  " Pk1" : Outport  Port=9
  " iAout" : Outport  Port=10

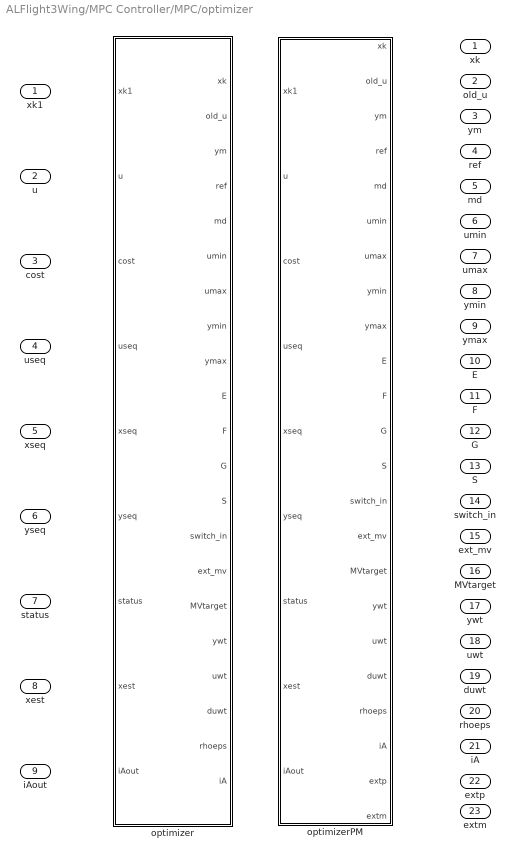
== system ALFlight3Wing/MPC Controller/MPC/optimizer ==
  "xk " : Inport
  "old_u " : Inport  Port=2
  "ym " : Inport  Port=3
  "ref " : Inport  Port=4
  "md " : Inport  Port=5
  "umin " : Inport  Port=6
  "umax " : Inport  Port=7
  "ymin " : Inport  Port=8
  "ymax " : Inport  Port=9
  "E " : Inport  Port=10
  "F " : Inport  Port=11
  "G " : Inport  Port=12
  "S " : Inport  Port=13
  "switch_in " : Inport  Port=14
  "ext_mv " : Inport  Port=15
  "MVtarget " : Inport  Port=16
  "ywt " : Inport  Port=17
  "uwt " : Inport  Port=18
  "duwt " : Inport  Port=19
  "rhoeps " : Inport  Port=20
  "iA " : Inport  Port=21
  extp : Inport  Port=22
  extm : Inport  Port=23
  optimizer : MATLAB Function  VariantControl=FixedHorizon
  optimizerPM : MATLAB Function  VariantControl=VariableHorizon
  " xk1" : Outport
  " u" : Outport  Port=2
  " cost" : Outport  Port=3
  " useq" : Outport  Port=4
  " xseq" : Outport  Port=5
  " yseq" : Outport  Port=6
  " status" : Outport  Port=7
  " xest" : Outport  Port=8
  " iAout" : Outport  Port=9

== matlab function ALFlight3Wing/MATLAB Function1 ==
  data: bestA output; uncertainty data_store_memory; savedInputs data_store_memory; savedOutputs data_store_memory; counts data_store_memory; currentState data_store_memory; in input; action data_store_memory; ABestGuess data_store_memory; useMPC data_store_memory; actionCount data_store_memory; allActions data_store_memory
function bestA= fcn10(in)
         coder.extrinsic('calcDynamics')
         coder.extrinsic('selectBayesianA')
         coder.extrinsic('chanceConstraintProgramming4')
global uncertainty
global savedInputs
global savedOutputs
global counts
global currentState
global action
global ABestGuess
global useMPC
global actionCount
global allActions
coder.extrinsic('assignin')
    bestA=zeros(4,1);
    numStates=11;
    numOutputs=11;
    if counts>10 && ~useMPC
        if  actionCount==2
        inputsT=savedInputs(:,1:counts)
        outputsT=savedOutputs(:,1:counts)
        deltaSEst=zeros(numOutputs,counts);
        states=inputsT(5:15,:)
        actions=inputsT(1:4,:)

        for i =1:size(inputsT,2)
            deltaSEst(:,i)=simulateNominal(states(:,i),actions(:,i));
        end

        trainingInputs=[actions;deltaSEst];
        trainingOutputs=(outputsT-inputsT(5:end,:))/.05

        assignin('base','ABestGuess',ABestGuess)
        %%create bootstrapped models
        Z=700;
        NET = cell(Z,1);
        error=zeros(Z,1)
        for i=1:Z
            %indices of samples used for bootstrapping. Randomly sampled with replacement
            bootSamples= randi(size(trainingInputs,2),size(trainingInputs,2),1);
            xBoot=zeros(15,counts);
            yBoot=zeros(11,counts);
            %Pick out samples from training inputs and outputs
            for b=1:size(trainingInputs,2)
                xBoot(:,b)=trainingInputs(:,bootSamples(b));
                yBoot(:,b)=trainingOutputs(:,bootSamples(b));
            end
            %All samples used for trainging and testing
            NET{i}=pinv(xBoot)'*yBoot';
            error(i)=sum(norm(NET{i}'*trainingInputs-trainingOutputs));
            %uncertainty=uncertainty+sum(sum(abs(ABestGuess-NET{i})))
 
        end
        
        [B,I] = mink(error,3);
        
        A=NET{I(1)}
        A=reshape(A,15,11)
        ABestGuess=A
        
            As=cat(3,NET{I(1)},NET{I(2)},NET{I(3)});
            AAverage=mean(As,3);
            Astd=std(As,[],3);
            uncertainty=sum(sum(Astd))

        [allActions]=chanceConstraintProgramming4(currentState,uncertainty,ABestGuess,{NET{I(1)},NET{I(2)},NET{I(3)}},action,trainingInputs(1:4,:))
        actionCount=1
        bestA=allActions(1:4)
        bestA=reshape(bestA,4,1)

        else
            bestA=allActions(5:8)
            bestA=reshape(bestA,4,1)
            actionCount=2

        end
    end

== matlab function ALFlight3Wing/MATLAB Function ==
  data: nextState output; state input; y output; action input; Ts input; time input; currentState data_store_memory; counts data_store_memory
function [nextState,y] = fcn2(state, action,Ts,time)
global currentState
Anominal=[-0.0220400000000000,0.00142200000000000,0,-32.1700000000000,0,0,0,0,0,0,0;
    -0.0575900000000000,-0.394300000000000,871,0,0,0,0,0,0,0,0;
    -9.50000000000000e-05,-0.00179300000000000,-0.546800000000000,0,0,0,0,0,0,0,0;
    0,0,1,0,0,0,0,0,0,0,0;
    0,0,0,0,-0.0639900000000000,0,-1,0.0369100000000000,0,0,0;
    0,0,0,0,-2.11100000000000,-0.504800000000000,0.193000000000000,0,0,0,0;
    0,0,0,0,0.773200000000000,0.0108700000000000,-0.179400000000000,0,0,0,0;
    0,0,0,0,0,1,0,0,0,0,0;
    0,0,0,0,0,0,1,0,0,0,0;
    1,0,0,0,0,0,0,0,0,0,0;
    0,1,0,0,0,0,0,0,0,0,0];
Bnominal=[0,1.91000000000000e-05,0,0;
    -18.5800000000000,0,0,0;
    -1.20000000000000,0,0,0;
    0,0,0,0;
    0,0,0,0.00839000000000000;
    0,0,0.184800000000000,0.105600000000000;
    0,0,-0.00869900000000000,-0.459100000000000;
    0,0,0,0;
    0,0,0,0;
    0,0,0,0;
    0,0,0,0];

Afault2=[-0.0220400000000000,0.00142200000000000,0,-32.1700000000000,0,0,0,0,0,0,0;
    -0.0575900000000000,-0.394300000000000,871,0,0,0,0,0,0,0,0;
    -9.50000000000000e-05,-0.00179300000000000,-0.546800000000000,0,0,0,0,0,0,0,0;
    0,0,1,0,0,0,0,0,0,0,0;
    0,0,0,0,0,-0.00110800000000000,-1,0.0369100000000000,0,0,0;
    0,0,0,0,-1.23500000000000,-0.481800000000000,0.0891100000000000,0,0,0,0;
    0,0,0,0,0,-0.0519300000000000,0,0,0,0,0;
    0,0,0,0,0,1,0,0,0,0,0;
    0,0,0,0,0,0,1,0,0,0,0;
    1,0,0,0,0,0,0,0,0,0,0;
    0,1,0,0,0,0,0,0,0,0,0];
Bfault2=[0,1.91000000000000e-05,0,0;
    -18.5800000000000,0,0,0;
    -1.20000000000000,0,0,0;
    0,0,0,0;
    0,0,0,0;
    0,0,0.187900000000000,0;
    0,0,0,0;
    0,0,0,0;
    0,0,0,0;
    0,0,0,0;
    0,0,0,0];

Afault1_2=[-0.0777422601610909,0.364315718281914,0,-49.5311012194985,0,0,0,0,0,0,0;
    0,-2.11693319505418,-8.082029025490,0,0,0,0,0,0,0,0;
    0.00516641602336364,-3.5543885272319,-2.926680000000,-2.37481704217243,0,0,0,0,0,0,0;
    0,0,1,0,0,0,0,0,0,0,0;
    0,0,0,0,-1.73568157299046,-0.00695689900121296,-246.715568807515,49.5311012194985,0,0,0;
    0,0,32.90144280000,31.3713331270978,-0.0210854784922154,-0.00633571574984461,0.00174212652554297,0,0,0,0;
    0,0,0,13.2100000000000,0.0233794202315124,-4.26083552968259e-05,-0.00576851579403181,0,0,0,0;
    0,0,0,0,0,1,0.0479459770467924,0,0,0,0;
    0,0,0,0,0,0,1,0,0,0,0;
    1,0,0,0,0,0,0,0,0,0,0;
    0,1,0,0,0,0,0,0,0,0,0].*.25
Bfault1_2=[0,0,0,0;
    -.11693319505418,0,0,0;
    -1.863280824027,0,0,0;
    0,0,0,0;
    0,0,0,-0.00412083182815909;
    0,0,0.00602442242634726,0.00602442242634726;
    0,0,0,-0.0221156677865658;
    0,0,0,0;0,0,0,0;0,0,0,0;0,0,0,0].*.25
 
Afault1=[-0.00470000000000000,-0.0107700000000000,0,-623300,0,0,0,0,0,0,0;
     -0.310000000000000,-0.253000000000000,16780000,-28300,0,0,0,0,0,0,0;
     0,0,-157900,264.600000000000,0,0,0,0,0,0,0;
     0,0,1,0,0,0,0,0,0,0,0;
     0,0,0,0,-0.0470000000000000,0,-16890000,620000,0,0,0;
     0,0,463000,-7797,-0.00160000000000000,-0.201300000000000,0.105500000000000,0,0,0,0;
     0,0,0,171900,0.000570000000000000,-0.00650000000000000,-157900,5833,0,0,0;
     0,0,0,0,0,1,0.0454100000000000,0,0,0,0;
     0,0,0,0,0,0,1,0,0,0,0;
     1,0,0,0,0,0,0,0,0,0,0;
     0,871,0,0,0,0,0,0,0,0,0];
 Bfault1=[0,0,0,0;
     13.3300000000000,0,0,0;
     -0.914700000000000,0,0,0;
     0,0,0,0;
     0,0,0,5.37700000000000;
     0,0,0.0670800000000000,0.0762900000000000;
     0,0,13.3200000000000,-0.289500000000000;
     0,0,0,0;
     0,0,0,0;
     0,0,0,0;
     0,0,0,0];
 
 
 Afault3=[-0.0220400000000000,0.00142200000000000,0,-32.1700000000000,0,0,0,0,0,0,0;-0.0575900000000000,-0.394300000000000,871,0,0,0,0,0,0,0,0;-9.50000000000000e-05,-0.00179300000000000,-0.546800000000000,0,0,0,0,0,0,0,0;0,0,1,0,0,0,0,0,0,0,0;0,0,0,0,-0.0639900000000000,0,-1,0.0369100000000000,0,0,0;0,0,0,0,-2.11100000000000,-0.504800000000000,0.193000000000000,0,0,0,0;0,0,0,0,0.773200000000000,0.0108700000000000,-0.179400000000000,0,0,0,0;0,0,0,0,0,1,0,0,0,0,0;0,0,0,0,0,0,1,0,0,0,0;1,0,0,0,0,0,0,0,0,0,0;0,1,0,0,0,0,0,0,0,0,0]
Bfault3=[0,1.91000000000000e-05,0,0;
    -18.5800000000000,0,0,0;
    -1.20000000000000,0,0,0;
    0,0,0,0;
    0,0,0,0.00839000000000000;
    0,0,0,0.105600000000000;
    0,0,0,-0.459100000000000;
    0,0,0,0;
    0,0,0,0;
    0,0,0,0;
    0,0,0,0]
 
 % C=[1,0,0,0,0,0,0,0,0,0,0;
%     0,0,0,1,0,0,0,0,0,0,0;
%     0,0,0,0,0,0,0,1,0,0,0;
%     0,0,0,0,0,0,0,0,1,0,0;
%     0,0,0,0,0,0,0,0,0,1,0;
%     0,0,0,0,0,0,0,0,0,0,1]
 %y=zeros(6,1);
deltaS=zeros(11,1)
 if time<30
     deltaS=Anominal*state*Ts+Bnominal*action*Ts;
     nextState=deltaS+state
    y=nextState
 else
     deltaS=Afault2*state*Ts+Bfault2*action*Ts
     nextState=deltaS+state
     y=nextState
 end
 currentState=y
end

== matlab function ALFlight3Wing/MATLAB Function2 ==
  data: error input; counts data_store_memory
function fcn(error)
global counts
if error>.01
counts=counts+1
end

== matlab function ALFlight3Wing/MATLAB Function3 ==
  data: outputs input; counts data_store_memory; savedOutputs data_store_memory
function saveDataOutputs(outputs)
global savedOutputs
global counts
if counts>0
savedOutputs(:,counts)=outputs
end
x=savedOutputs

== matlab function ALFlight3Wing/State space model ==
  data: state input; nextState output; action input; Ts input; time input; action output; y output
function [nextState,action,y] = fcn(state, action, Ts,time)
Anominal=[-0.0220400000000000,0.00142200000000000,0,-32.1700000000000,0,0,0,0,0,0,0,0;-0.0575900000000000,-0.394300000000000,871,0,0,0,0,0,0,0,0,0;-9.50000000000000e-05,-0.00179300000000000,-0.546800000000000,0,0,0,0,0,0,0,0,0;0,0,1,0,0,0,0,0,0,0,0,0;0,0,0,0,-0.0639900000000000,0,-1,0.0369100000000000,0,0,0,0;0,0,0,0,-2.11100000000000,-0.504800000000000,0.193000000000000,0,0,0,0,0;0,0,0,0,0.773200000000000,0.0108700000000000,-0.179400000000000,0,0,0,0,0;0,0,0,0,0,1,0,0,0,0,0,0;0,0,0,0,0,0,1,0,0,0,0,0;1,0,0,0,0,0,0,0,0,0,0,0;0,1,0,0,0,0,0,0,0,0,0,0;0,0,0,0,0,0,0,0,0,0,0,0]
Bnominal=[0,1.91000000000000e-05,0,0;-18.5800000000000,0,0,0;-1.20000000000000,0,0,0;0,0,0,0;0,0,0,0.00839000000000000;0,0,0.184800000000000,0.105600000000000;0,0,-0.00869900000000000,-0.459100000000000;0,0,0,0;0,0,0,0;0,0,0,0;0,0,0,0;0,0,0,0]

Afault2=[-0.0220400000000000,0.00142200000000000,0,-32.1700000000000,0,0,0,0,0,0,0;
    -0.0575900000000000,-0.394300000000000,871,0,0,0,0,0,0,0,0;
    -9.50000000000000e-05,-0.00179300000000000,-0.546800000000000,0,0,0,0,0,0,0,0;
    0,0,1,0,0,0,0,0,0,0,0;
    0,0,0,0,0,-0.00110800000000000,-1,0.0369100000000000,0,0,0;
    0,0,0,0,-1.23500000000000,-0.481800000000000,0.0891100000000000,0,0,0,0;
    0,0,0,0,0,-0.0519300000000000,0,0,0,0,0;
    0,0,0,0,0,1,0,0,0,0,0;
    0,0,0,0,0,0,1,0,0,0,0;
    1,0,0,0,0,0,0,0,0,0,0;
    0,1,0,0,0,0,0,0,0,0,0];
Bfault2=[0,1.91000000000000e-05,0,0;
    -18.5800000000000,0,0,0;
    -1.20000000000000,0,0,0;
    0,0,0,0;
    0,0,0,0;
    0,0,0.187900000000000,0;
    0,0,0,0;
    0,0,0,0;
    0,0,0,0;
    0,0,0,0;
    0,0,0,0];
     
 Afault1=[-0.00470000000000000,-0.0107700000000000,0,-623300,0,0,0,0,0,0,0;
     -0.310000000000000,-0.253000000000000,16780000,-28300,0,0,0,0,0,0,0;
     0,0,-157900,264.600000000000,0,0,0,0,0,0,0;
     0,0,1,0,0,0,0,0,0,0,0;
     0,0,0,0,-0.0470000000000000,0,-16890000,620000,0,0,0;
     0,0,463000,-7797,-0.00160000000000000,-0.201300000000000,0.105500000000000,0,0,0,0;
     0,0,0,171900,0.000570000000000000,-0.00650000000000000,-157900,5833,0,0,0;
     0,0,0,0,0,1,0.0454100000000000,0,0,0,0;
     0,0,0,0,0,0,1,0,0,0,0;
     1,0,0,0,0,0,0,0,0,0,0;
     0,1,0,0,0,0,0,0,0,0,0];
 Bfault1=[0,0,0,0;
     13.3300000000000,0,0,0;
     -0.914700000000000,0,0,0;
     0,0,0,0;
     0,0,0,5.37700000000000;
     0,0,0.0670800000000000,0.0762900000000000;
     0,0,13.3200000000000,-0.289500000000000;
     0,0,0,0;
     0,0,0,0;
     0,0,0,0;
     0,0,0,0];
C=[1,0,0,0,0,0,0,0,0,0,0,0;0,0,0,1,0,0,0,0,0,0,0,0;0,0,0,0,0,0,0,1,0,0,0,0;0,0,0,0,0,0,0,0,1,0,0,0;0,0,0,0,0,0,0,0,0,1,0,0;0,0,0,0,0,0,0,0,0,0,1,0]
y=zeros(6,1);
deltaS=zeros(12,1)
 if time<20
     deltaS=Anominal*state*.05+Bnominal*action*.05;
    nextState=(deltaS+state);
    y=C*nextState;
 else
     nextState=zeros(12,1)
%     deltaS=Afault2*state*Ts+Bfault2*action*Ts;
%     nextState=(deltaS+state);
%     y=C*nextState;
end
end

== matlab function ALFlight3Wing/MATLAB Function4 ==
  data: a output; actionMPC input; actionAL input; counts data_store_memory; uncertainty data_store_memory; useMPC data_store_memory; ABestGuess data_store_memory
function a = switching(actionMPC,actionAL)
coder.extrinsic('evalin')
coder.extrinsic('set_param')
global counts
global uncertainty
global useMPC
global ABestGuess

Anominal=[-0.0220400000000000,0.00142200000000000,0,-32.1700000000000,0,0,0,0,0,0,0;
    -0.0575900000000000,-0.394300000000000,871,0,0,0,0,0,0,0,0;
    -9.50000000000000e-05,-0.00179300000000000,-0.546800000000000,0,0,0,0,0,0,0,0;
    0,0,1,0,0,0,0,0,0,0,0;
    0,0,0,0,-0.0639900000000000,0,-1,0.0369100000000000,0,0,0;
    0,0,0,0,-2.11100000000000,-0.504800000000000,0.193000000000000,0,0,0,0;
    0,0,0,0,0.773200000000000,0.0108700000000000,-0.179400000000000,0,0,0,0;
    0,0,0,0,0,1,0,0,0,0,0;
    0,0,0,0,0,0,1,0,0,0,0;
    1,0,0,0,0,0,0,0,0,0,0;
    0,1,0,0,0,0,0,0,0,0,0];
Bnominal=[0,1.91000000000000e-05,0,0;
    -18.5800000000000,0,0,0;
    -1.20000000000000,0,0,0;
    0,0,0,0;
    0,0,0,0.00839000000000000;
    0,0,0.184800000000000,0.105600000000000;
    0,0,-0.00869900000000000,-0.459100000000000;
    0,0,0,0;
    0,0,0,0;
    0,0,0,0;
    0,0,0,0];



a=actionMPC;
if counts>10 && ~useMPC
    a=actionAL;
end
if uncertainty<5
    useMPC=true
    
    ABestGuess(abs(ABestGuess)<1e-7)=0
    Af=ABestGuess(5:15,:)*Anominal
    AfU=Af([1 2 3 4 5 6 7 8 9 11],[1 2 3 4 5 6 7 8 9 11])
    Bf= ABestGuess(1:4,:)'+ABestGuess(5:15,:)'*Bnominal
    BfU=Bf([1 2 3 4 5 6 7 8 9 11],:)

    Af2=evalin('base','Af2')
    Bf2=evalin('base','Bf2')

    
    
    set_param('ALFlight3Wing/ConstantA','Value','Af2')
    set_param('ALFlight3Wing/ConstantB','Value','Bf2')

end
%     fault1MPC.Model.Plant.A=A
%     fault1MPC.Model.Plant.B=B
%     
%     fault2MPC.Model.Plant.A=A
%     fault2MPC.Model.Plant.B=B
%     
%     fault3MPC.Model.Plant.A=A
%     fault3MPC.Model.Plant.B=B
% set_param('testMPC/MPCController1','mpcobj','fault2MPC')

% a=actionMPC;
% if time>1000
%     a=actionAL;
% end

== matlab function ALFlight3Wing/MATLAB Function5 ==
  data: inputs input; savedInputs data_store_memory; counts data_store_memory
function saveDataInputs(inputs)
global savedInputs
global counts
if counts>0
savedInputs(:,counts)=inputs
end
x=savedInputs
